simulink model "ecg_qrs_detector"  (R2021a)
settings: Solver=FixedStepDiscrete  StartTime=0.0  StopTime=5.0  FixedStep=.004  RelTol=1e-3
undefined symbols (not defined in the file): sampleTime, THRESHOLD_ONE, THRESHOLD_TWO
libraries: simulink x4, dspstat3 x2
settings Model: Creator=wallyproenza  LastModifiedBy=wallyproenza

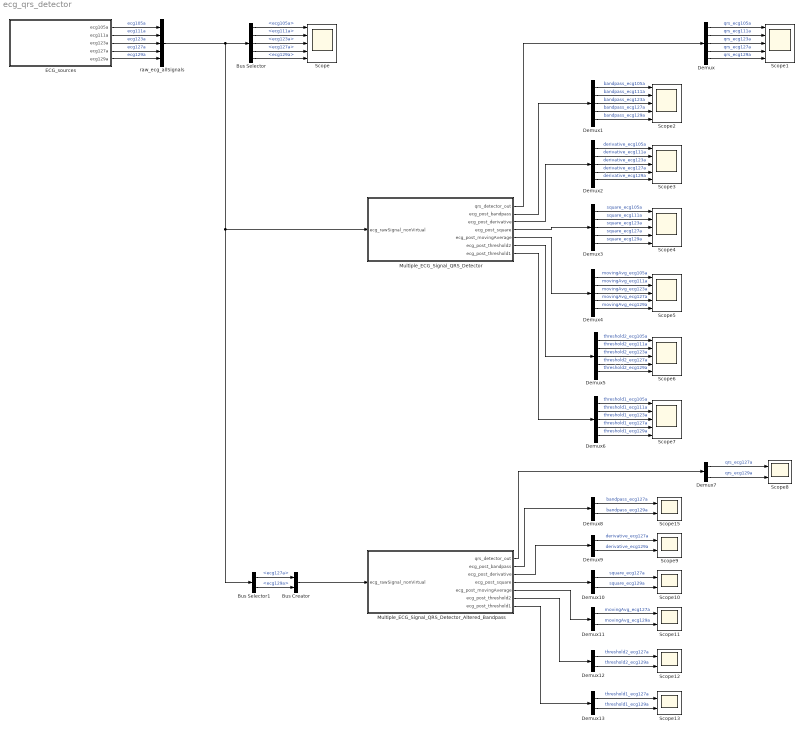
== system ecg_qrs_detector ==
  Bus Creator : BusCreator  Inputs=2  OutDataTypeStr=Bus: bottom2_raw_ecg_signals  NonVirtualBus=on
  Bus Selector : BusSelector  OutputSignals=ecg105a,ecg111a,ecg123a,ecg127a,ecg129a
  Bus Selector1 : BusSelector  OutputSignals=ecg127a,ecg129a
  Demux{,1..6} (7 alike) : Demux  Outputs=5
  Demux{7..13} (7 alike) : Demux  Outputs=2
  ECG_sources : Subsystem
  "Multiple_ECG_Signal_QRS_Detector " : Subsystem  TreatAsAtomicUnit=on
  Multiple_ECG_Signal_QRS_Detector_Altered_Bandpass : Subsystem  TreatAsAtomicUnit=on
  Scope{,1..7} (8 alike) : Scope  NumInputPorts=5
  Scope{8..13,15} (7 alike) : Scope  NumInputPorts=2
  raw_ecg_allSignals : BusCreator  Inputs=5  OutDataTypeStr=Bus: raw_ecg_signals  NonVirtualBus=on
  wires:
  ECG_sources/1(ecg105a) -> raw_ecg_allSignals/1  "ecg105a"
  ECG_sources/2(ecg111a) -> raw_ecg_allSignals/2  "ecg111a"
  ECG_sources/3(ecg123a) -> raw_ecg_allSignals/3  "ecg123a"
  ECG_sources/4(ecg127a) -> raw_ecg_allSignals/4  "ecg127a"
  ECG_sources/5(ecg129a) -> raw_ecg_allSignals/5  "ecg129a"
  raw_ecg_allSignals/1 -> "Multiple_ECG_Signal_QRS_Detector "/1(ecg_rawSignal_nonVirtual), Bus Selector1/1, Bus Selector/1
  Bus Selector/1 -> Scope/1  "<ecg105a>"
  Bus Selector/2 -> Scope/2  "<ecg111a>"
  Bus Selector/3 -> Scope/3  "<ecg123a>"
  Bus Selector/4 -> Scope/4  "<ecg127a>"
  Bus Selector/5 -> Scope/5  "<ecg129a>"
  "Multiple_ECG_Signal_QRS_Detector "/1(qrs_detector_out) -> Demux/1
  Demux/1 -> Scope1/1  "qrs_ecg105a"
  Demux/2 -> Scope1/2  "qrs_ecg111a"
  Demux/3 -> Scope1/3  "qrs_ecg123a"
  Demux/4 -> Scope1/4  "qrs_ecg127a"
  Demux/5 -> Scope1/5  "qrs_ecg129a"
  Demux1/5 -> Scope2/5  "bandpass_ecg129a"
  Demux1/2 -> Scope2/2  "bandpass_ecg111a"
  Demux1/4 -> Scope2/4  "bandpass_ecg127a"
  Demux1/1 -> Scope2/1  "bandpass_ecg105a"
  Demux1/3 -> Scope2/3  "bandpass_ecg123a"
  "Multiple_ECG_Signal_QRS_Detector "/2(ecg_post_bandpass) -> Demux1/1
  Demux2/1 -> Scope3/1  "derivative_ecg105a"
  Demux2/2 -> Scope3/2  "derivative_ecg111a"
  Demux2/3 -> Scope3/3  "derivative_ecg123a"
  Demux2/4 -> Scope3/4  "derivative_ecg127a"
  Demux2/5 -> Scope3/5  "derivative_ecg129a"
  "Multiple_ECG_Signal_QRS_Detector "/3(ecg_post_derivative) -> Demux2/1
  Demux3/1 -> Scope4/1  "square_ecg105a"
  Demux3/2 -> Scope4/2  "square_ecg111a"
  Demux3/3 -> Scope4/3  "square_ecg123a"
  Demux3/4 -> Scope4/4  "square_ecg127a"
  Demux3/5 -> Scope4/5  "square_ecg129a"
  "Multiple_ECG_Signal_QRS_Detector "/4(ecg_post_square) -> Demux3/1
  Demux4/1 -> Scope5/1  "movingAvg_ecg105a"
  Demux4/2 -> Scope5/2  "movingAvg_ecg111a"
  Demux4/3 -> Scope5/3  "movingAvg_ecg123a"
  Demux4/4 -> Scope5/4  "movingAvg_ecg127a"
  Demux4/5 -> Scope5/5  "movingAvg_ecg129a"
  "Multiple_ECG_Signal_QRS_Detector "/5(ecg_post_movingAverage) -> Demux4/1
  Demux5/1 -> Scope6/1  "threshold2_ecg105a"
  Demux5/2 -> Scope6/2  "threshold2_ecg111a"
  Demux5/3 -> Scope6/3  "threshold2_ecg123a"
  Demux5/4 -> Scope6/4  "threshold2_ecg127a"
  Demux5/5 -> Scope6/5  "threshold2_ecg129a"
  "Multiple_ECG_Signal_QRS_Detector "/6(ecg_post_threshold2) -> Demux5/1
  Demux6/1 -> Scope7/1  "threshold1_ecg105a"
  Demux6/2 -> Scope7/2  "threshold1_ecg111a"
  Demux6/3 -> Scope7/3  "threshold1_ecg123a"
  Demux6/4 -> Scope7/4  "threshold1_ecg127a"
  Demux6/5 -> Scope7/5  "threshold1_ecg129a"
  "Multiple_ECG_Signal_QRS_Detector "/7(ecg_post_threshold1) -> Demux6/1
  Multiple_ECG_Signal_QRS_Detector_Altered_Bandpass/1(qrs_detector_out) -> Demux7/1
  Demux7/1 -> Scope8/1  "qrs_ecg127a"
  Demux7/2 -> Scope8/2  "qrs_ecg129a"
  Demux13/1 -> Scope13/1  "threshold1_ecg127a"
  Demux12/2 -> Scope12/2  "threshold2_ecg129a"
  Multiple_ECG_Signal_QRS_Detector_Altered_Bandpass/7(ecg_post_threshold1) -> Demux13/1
  Demux8/1 -> Scope15/1  "bandpass_ecg127a"
  Demux8/2 -> Scope15/2  "bandpass_ecg129a"
  Demux13/2 -> Scope13/2  "threshold1_ecg129a"
  Demux11/2 -> Scope11/2  "movingAvg_ecg129a"
  Demux11/1 -> Scope11/1  "movingAvg_ecg127a"
  Demux9/2 -> Scope9/2  "derivative_ecg129a"
  Demux12/1 -> Scope12/1  "threshold2_ecg127a"
  Multiple_ECG_Signal_QRS_Detector_Altered_Bandpass/4(ecg_post_square) -> Demux10/1
  Demux10/2 -> Scope10/2  "square_ecg129a"
  Multiple_ECG_Signal_QRS_Detector_Altered_Bandpass/5(ecg_post_movingAverage) -> Demux11/1
  Multiple_ECG_Signal_QRS_Detector_Altered_Bandpass/2(ecg_post_bandpass) -> Demux8/1
  Demux10/1 -> Scope10/1  "square_ecg127a"
  Multiple_ECG_Signal_QRS_Detector_Altered_Bandpass/3(ecg_post_derivative) -> Demux9/1
  Multiple_ECG_Signal_QRS_Detector_Altered_Bandpass/6(ecg_post_threshold2) -> Demux12/1
  Demux9/1 -> Scope9/1  "derivative_ecg127a"
  Bus Selector1/2 -> Bus Creator/2  "<ecg129a>"
  Bus Selector1/1 -> Bus Creator/1  "<ecg127a>"
  Bus Creator/1 -> Multiple_ECG_Signal_QRS_Detector_Altered_Bandpass/1(ecg_rawSignal_nonVirtual)

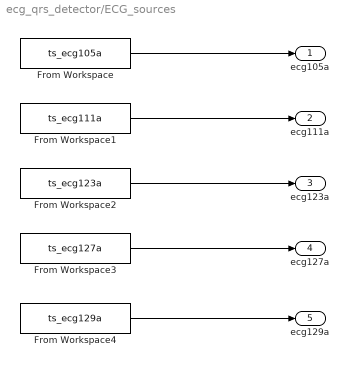
== system ecg_qrs_detector/ECG_sources ==
  From Workspace : FromWorkspace  VariableName=ts_ecg105a
  From Workspace1 : FromWorkspace  VariableName=ts_ecg111a
  From Workspace2 : FromWorkspace  VariableName=ts_ecg123a
  From Workspace3 : FromWorkspace  VariableName=ts_ecg127a
  From Workspace4 : FromWorkspace  VariableName=ts_ecg129a
  ecg105a : Outport
  ecg111a : Outport  Port=2
  ecg123a : Outport  Port=3
  ecg127a : Outport  Port=4
  ecg129a : Outport  Port=5
  wires:
  From Workspace3/1 -> ecg127a/1
  From Workspace1/1 -> ecg111a/1
  From Workspace2/1 -> ecg123a/1
  From Workspace4/1 -> ecg129a/1
  From Workspace/1 -> ecg105a/1

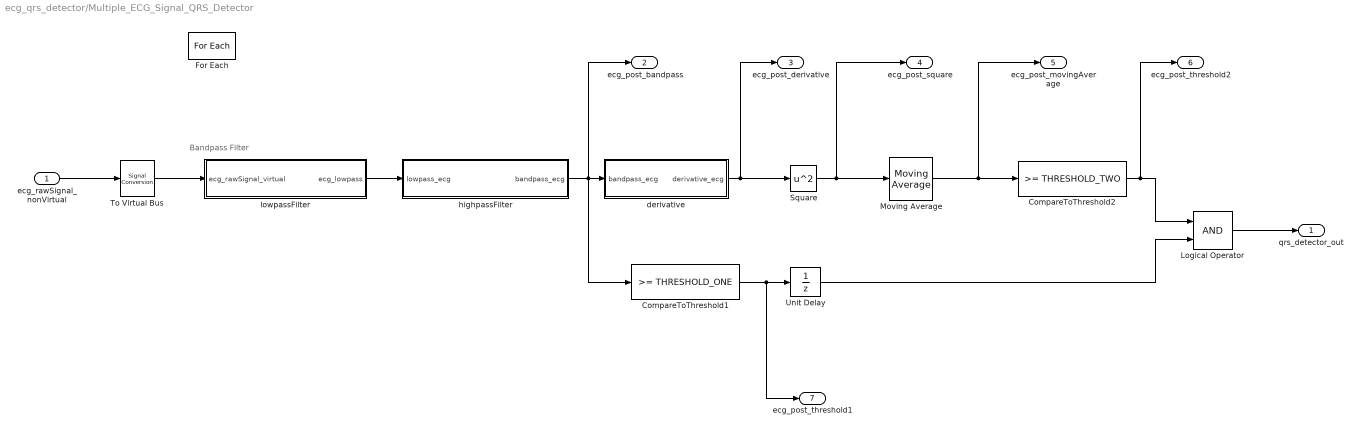
== system ecg_qrs_detector/Multiple_ECG_Signal_QRS_Detector  ==
  note: Bandpass Filter
  ecg_rawSignal_nonVirtual : Inport  Partition=on  PartitionDimension=1  PartitionWidth=1  PartitionOffset=0
  CompareToThreshold1 : simulink/Logic and Bit Operations/Compare To Constant  relop=>=  const=THRESHOLD_ONE  OutDataTypeStr=boolean
  CompareToThreshold2 : simulink/Logic and Bit Operations/Compare To Constant  relop=>=  const=THRESHOLD_TWO  OutDataTypeStr=boolean
  For Each : ForEach  DisableCoverage=on
  Logical Operator : Logic  IconShape=distinctive  AllPortsSameDT=off  OutDataTypeStr=boolean
  Moving Average : dspstat3/Moving Average  Method=Sliding window  ForgettingFactorPort=off  SpecifyWindowLength=on  WindowLength=38  ForgettingFactor=0.9  SimulateUsing=Code generation
  Square : Math  Operator=square  SaturateOnIntegerOverflow=on
  To Virtual Bus : SignalConversion  ConversionOutput=Virtual bus  OverrideOpt=off
  Unit Delay : UnitDelay  SampleTime=-1  HasFrameUpgradeWarning=on
  derivative : Subsystem
  highpassFilter : Subsystem
  lowpassFilter : Subsystem
  qrs_detector_out : Outport  ConcatenationDimension=1
  ecg_post_bandpass : Outport  Port=2  ConcatenationDimension=1
  ecg_post_derivative : Outport  Port=3  ConcatenationDimension=1
  ecg_post_square : Outport  Port=4  ConcatenationDimension=1
  ecg_post_movingAverage : Outport  Port=5  ConcatenationDimension=1
  ecg_post_threshold2 : Outport  Port=6  ConcatenationDimension=1
  ecg_post_threshold1 : Outport  Port=7  ConcatenationDimension=1
  wires:
  highpassFilter/1(bandpass_ecg) -> derivative/1(bandpass_ecg), CompareToThreshold1/1, ecg_post_bandpass/1
  Moving Average/1 -> ecg_post_movingAverage/1, CompareToThreshold2/1
  derivative/1(derivative_ecg) -> ecg_post_derivative/1, Square/1
  CompareToThreshold2/1 -> Logical Operator/1, ecg_post_threshold2/1
  Unit Delay/1 -> Logical Operator/2
  CompareToThreshold1/1 -> ecg_post_threshold1/1, Unit Delay/1
  Square/1 -> Moving Average/1, ecg_post_square/1
  Logical Operator/1 -> qrs_detector_out/1
  To Virtual Bus/1 -> lowpassFilter/1(ecg_rawSignal_virtual)
  ecg_rawSignal_nonVirtual/1 -> To Virtual Bus/1
  lowpassFilter/1(ecg_lowpass) -> highpassFilter/1(lowpass_ecg)

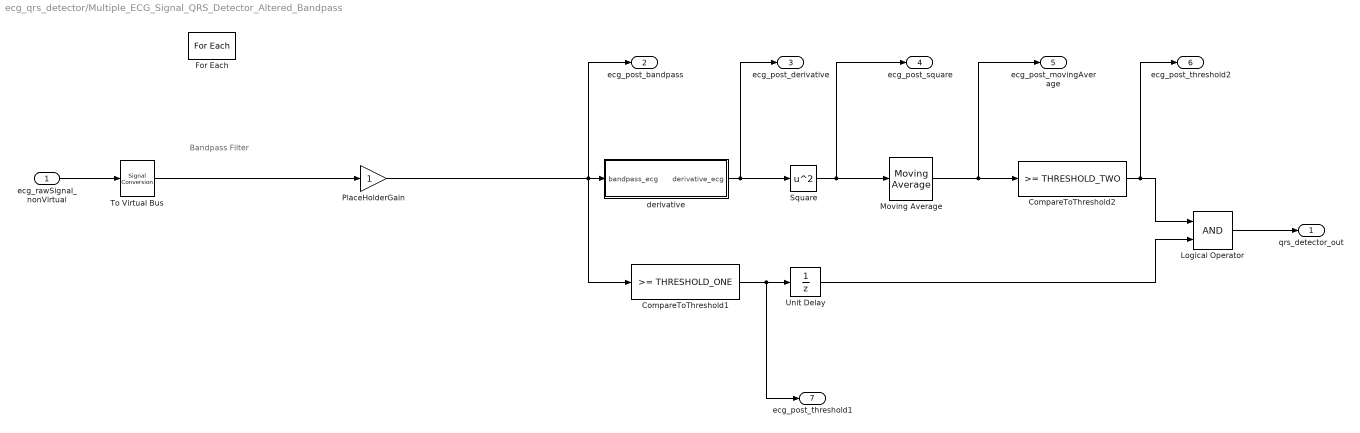
== system ecg_qrs_detector/Multiple_ECG_Signal_QRS_Detector_Altered_Bandpass ==
  note: Bandpass Filter
  ecg_rawSignal_nonVirtual : Inport  Partition=on  PartitionDimension=1  PartitionWidth=1  PartitionOffset=0
  CompareToThreshold1 : simulink/Logic and Bit Operations/Compare To Constant  relop=>=  const=THRESHOLD_ONE  OutDataTypeStr=boolean
  CompareToThreshold2 : simulink/Logic and Bit Operations/Compare To Constant  relop=>=  const=THRESHOLD_TWO  OutDataTypeStr=boolean
  For Each : ForEach  DisableCoverage=on
  Logical Operator : Logic  IconShape=distinctive  AllPortsSameDT=off  OutDataTypeStr=boolean
  Moving Average : dspstat3/Moving Average  Method=Sliding window  ForgettingFactorPort=off  SpecifyWindowLength=on  WindowLength=38  ForgettingFactor=0.9  SimulateUsing=Code generation
  PlaceHolderGain : Gain
  Square : Math  Operator=square  SaturateOnIntegerOverflow=on
  To Virtual Bus : SignalConversion  ConversionOutput=Virtual bus  OverrideOpt=off
  Unit Delay : UnitDelay  SampleTime=-1  HasFrameUpgradeWarning=on
  derivative : Subsystem
  qrs_detector_out : Outport  ConcatenationDimension=1
  ecg_post_bandpass : Outport  Port=2  ConcatenationDimension=1
  ecg_post_derivative : Outport  Port=3  ConcatenationDimension=1
  ecg_post_square : Outport  Port=4  ConcatenationDimension=1
  ecg_post_movingAverage : Outport  Port=5  ConcatenationDimension=1
  ecg_post_threshold2 : Outport  Port=6  ConcatenationDimension=1
  ecg_post_threshold1 : Outport  Port=7  ConcatenationDimension=1
  wires:
  ecg_rawSignal_nonVirtual/1 -> To Virtual Bus/1
  Moving Average/1 -> ecg_post_movingAverage/1, CompareToThreshold2/1
  derivative/1(derivative_ecg) -> ecg_post_derivative/1, Square/1
  CompareToThreshold2/1 -> Logical Operator/1, ecg_post_threshold2/1
  Unit Delay/1 -> Logical Operator/2
  CompareToThreshold1/1 -> ecg_post_threshold1/1, Unit Delay/1
  Square/1 -> Moving Average/1, ecg_post_square/1
  Logical Operator/1 -> qrs_detector_out/1
  To Virtual Bus/1 -> PlaceHolderGain/1
  PlaceHolderGain/1 -> CompareToThreshold1/1, derivative/1(bandpass_ecg), ecg_post_bandpass/1

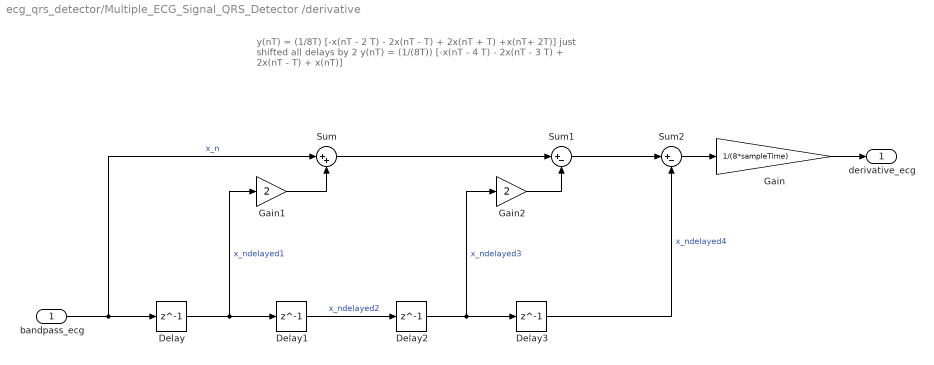
== system ecg_qrs_detector/Multiple_ECG_Signal_QRS_Detector /derivative ==
  note: y(nT) = (1/8T) [-x(nT - 2 T) - 2x(nT - T) + 2x(nT + T) +x(nT+ 2T)]
      |
      | just shifted all delays by 2
      |
      | y(nT) = (1/(8T)) [-x(nT - 4 T) - 2x(nT - 3 T) + 2x(nT - T) + x(nT)]
  bandpass_ecg : Inport
  Delay{,1..3} (4 alike) : Delay  DelayLength=1  InitialCondition=0
  Gain : Gain  Gain=1/(8*sampleTime)
  Gain1 : Gain  Gain=2
  Gain2 : Gain  Gain=2
  Sum : Sum  Inputs=|++
  Sum1 : Sum  Inputs=|+-
  Sum2 : Sum  Inputs=|+-
  derivative_ecg : Outport
  wires:
  Gain/1 -> derivative_ecg/1
  bandpass_ecg/1 -> Sum/1, Delay/1  "x_n"
  Delay/1 -> Gain1/1, Delay1/1  "x_ndelayed1"
  Delay1/1 -> Delay2/1  "x_ndelayed2"
  Delay2/1 -> Gain2/1, Delay3/1  "x_ndelayed3"
  Delay3/1 -> Sum2/2  "x_ndelayed4"
  Gain1/1 -> Sum/2
  Gain2/1 -> Sum1/2
  Sum/1 -> Sum1/1
  Sum1/1 -> Sum2/1
  Sum2/1 -> Gain/1

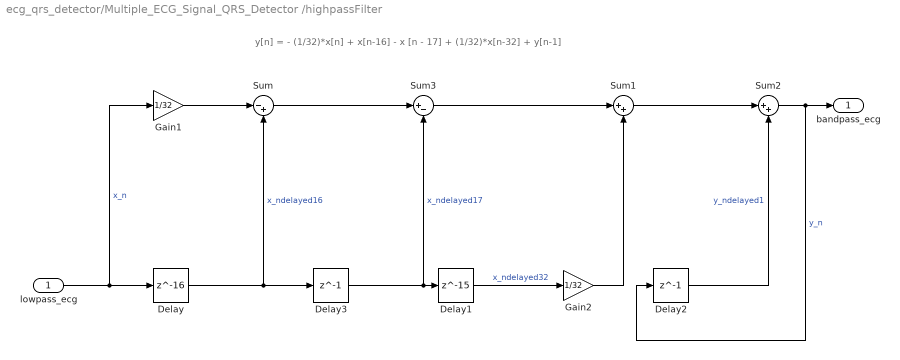
== system ecg_qrs_detector/Multiple_ECG_Signal_QRS_Detector /highpassFilter ==
  note: y[n] = - (1/32)*x[n] + x[n-16] - x [n - 17] + (1/32)*x[n-32] + y[n-1]
  lowpass_ecg : Inport
  Delay : Delay  DelayLength=16  InitialCondition=0
  Delay1 : Delay  DelayLength=15  InitialCondition=0
  Delay2 : Delay  DelayLength=1  InitialCondition=0
  Delay3 : Delay  DelayLength=1  InitialCondition=0
  Gain1 : Gain  Gain=1/32
  Gain2 : Gain  Gain=1/32
  Sum : Sum  Inputs=|-+
  Sum1 : Sum  Inputs=|++
  Sum2 : Sum  Inputs=|++
  Sum3 : Sum  Inputs=|+-
  bandpass_ecg : Outport
  wires:
  lowpass_ecg/1 -> Gain1/1, Delay/1  "x_n"
  Delay/1 -> Delay3/1, Sum/2  "x_ndelayed16"
  Delay1/1 -> Gain2/1  "x_ndelayed32"
  Sum1/1 -> Sum2/1
  Delay2/1 -> Sum2/2  "y_ndelayed1"
  Sum2/1 -> Delay2/1, bandpass_ecg/1  "y_n"
  Gain1/1 -> Sum/1
  Delay3/1 -> Delay1/1, Sum3/2  "x_ndelayed17"
  Sum/1 -> Sum3/1
  Sum3/1 -> Sum1/1
  Gain2/1 -> Sum1/2

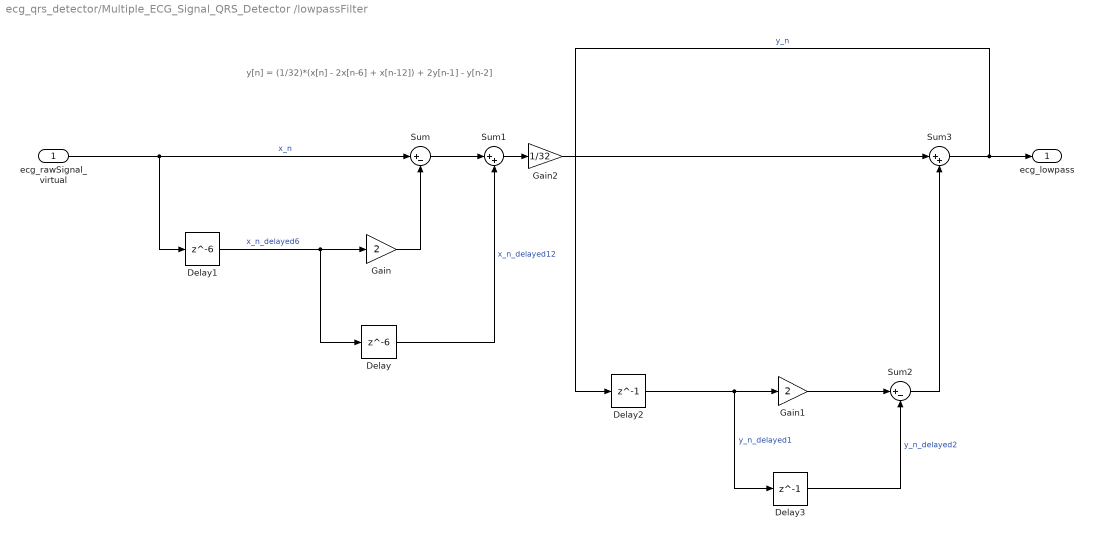
== system ecg_qrs_detector/Multiple_ECG_Signal_QRS_Detector /lowpassFilter ==
  note: y[n] = (1/32)*(x[n] - 2x[n-6] + x[n-12]) + 2y[n-1] - y[n-2]
  ecg_rawSignal_virtual : Inport
  Delay : Delay  DelayLength=6  InitialCondition=0
  Delay1 : Delay  DelayLength=6  InitialCondition=0
  Delay2 : Delay  DelayLength=1  InitialCondition=0
  Delay3 : Delay  DelayLength=1  InitialCondition=0
  Gain : Gain  Gain=2
  Gain1 : Gain  Gain=2
  Gain2 : Gain  Gain=1/32
  Sum : Sum  Inputs=|+-
  Sum1 : Sum  Inputs=|++
  Sum2 : Sum  Inputs=|+-
  Sum3 : Sum  Inputs=|++
  ecg_lowpass : Outport
  wires:
  ecg_rawSignal_virtual/1 -> Delay1/1, Sum/1  "x_n"
  Delay1/1 -> Gain/1, Delay/1  "x_n_delayed6"
  Gain/1 -> Sum/2
  Delay/1 -> Sum1/2  "x_n_delayed12"
  Sum/1 -> Sum1/1
  Sum1/1 -> Gain2/1
  Delay2/1 -> Delay3/1, Gain1/1  "y_n_delayed1"
  Gain1/1 -> Sum2/1
  Delay3/1 -> Sum2/2  "y_n_delayed2"
  Sum2/1 -> Sum3/2
  Sum3/1 -> ecg_lowpass/1, Delay2/1  "y_n"
  Gain2/1 -> Sum3/1

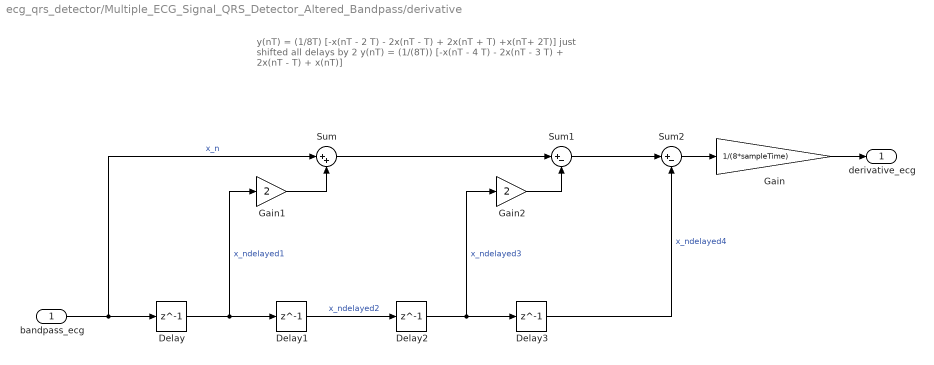
== system ecg_qrs_detector/Multiple_ECG_Signal_QRS_Detector_Altered_Bandpass/derivative ==
  note: y(nT) = (1/8T) [-x(nT - 2 T) - 2x(nT - T) + 2x(nT + T) +x(nT+ 2T)]
      |
      | just shifted all delays by 2
      |
      | y(nT) = (1/(8T)) [-x(nT - 4 T) - 2x(nT - 3 T) + 2x(nT - T) + x(nT)]
  bandpass_ecg : Inport
  Delay{,1..3} (4 alike) : Delay  DelayLength=1  InitialCondition=0
  Gain : Gain  Gain=1/(8*sampleTime)
  Gain1 : Gain  Gain=2
  Gain2 : Gain  Gain=2
  Sum : Sum  Inputs=|++
  Sum1 : Sum  Inputs=|+-
  Sum2 : Sum  Inputs=|+-
  derivative_ecg : Outport
  wires:
  Gain/1 -> derivative_ecg/1
  bandpass_ecg/1 -> Sum/1, Delay/1  "x_n"
  Delay/1 -> Gain1/1, Delay1/1  "x_ndelayed1"
  Delay1/1 -> Delay2/1  "x_ndelayed2"
  Delay2/1 -> Gain2/1, Delay3/1  "x_ndelayed3"
  Delay3/1 -> Sum2/2  "x_ndelayed4"
  Gain1/1 -> Sum/2
  Gain2/1 -> Sum1/2
  Sum/1 -> Sum1/1
  Sum1/1 -> Sum2/1
  Sum2/1 -> Gain/1
